simulink library "libbha_kinematic"  (R2015b)
settings: Solver=FixedStepDiscrete  StartTime=0.0  StopTime=Inf  FixedStep=0.004  RelTol=1e-3
PostLoadFcn:
  | , if any(exist('dsrtsu_mdlpostloadfcn', 'file') == [2, 3, 6]), try dsrtsu_mdlpostloadfcn('Execute', bdroot); catch fprintf('Error in PostLoadFcn (dsrtsu_mdlpostloadfcn) for model "%s":\n %s\n', bdroot, lasterr); end, end,
undefined symbols (not defined in the file or in its folder): BHA, BHASIM
libraries: libbha_kinematic x14
(part 1 of 3)
settings Model: DSRTSU_INTERNAL_RTI_VER=470  DSRTSU_INTERNAL_RTI_TYPE=rti1007  DSRTSU_INTERNAL_RTIFPGA=60  Creator=Falkenhahn  LastModifiedBy=isysfalkenhahn
settings DataIOCC: SaveFormat=Array
settings OptimizationCC: BlockReduction=off  OptimizeBlockIOStorage=off  BufferReuse=off  GlobalBufferReuse=off  ExpressionFolding=off  LocalBlockOutputs=off
settings DebuggingCC: UnderspecifiedInitializationDetection=Classic  MergeDetectMultiDrivingBlocksExec=none  SolverPrmCheckMsg=warning
settings HardwareCC: ProdBitPerPointer=32  ProdLargestAtomicFloat=None  ProdEndianess=BigEndian  ProdWordSize=32  ProdHWDeviceType=Generic->Custom  TargetIntDivRoundTo=Zero  TargetEndianess=BigEndian  TargetHWDeviceType=Generic->Custom
settings RTWCC: SystemTargetFile=rti1007.tlc  MakeCommand=make_rti  TemplateMakefile=rti1007.tmf  Description=dSPACE DS1007 Hardware Platform
settings STFCustomTargetCC: ParMdlRefBuildCompliant=on  ConcurrentExecutionCompliant=off  MatFileLogging=on  SystemTargetFile=rti1007.tlc
settings GRTTargetCC: CompOptLevelCompliant=off  ConcurrentExecutionCompliant=off  GeneratePreprocessorConditionals=Disable all  CombineOutputUpdateFcns=off  GRTInterface=on  UseToolchainInfoCompliant=off  ExtModeMexFile=noextcomm
settings ConfigComp: CovModelRefEnable=Off

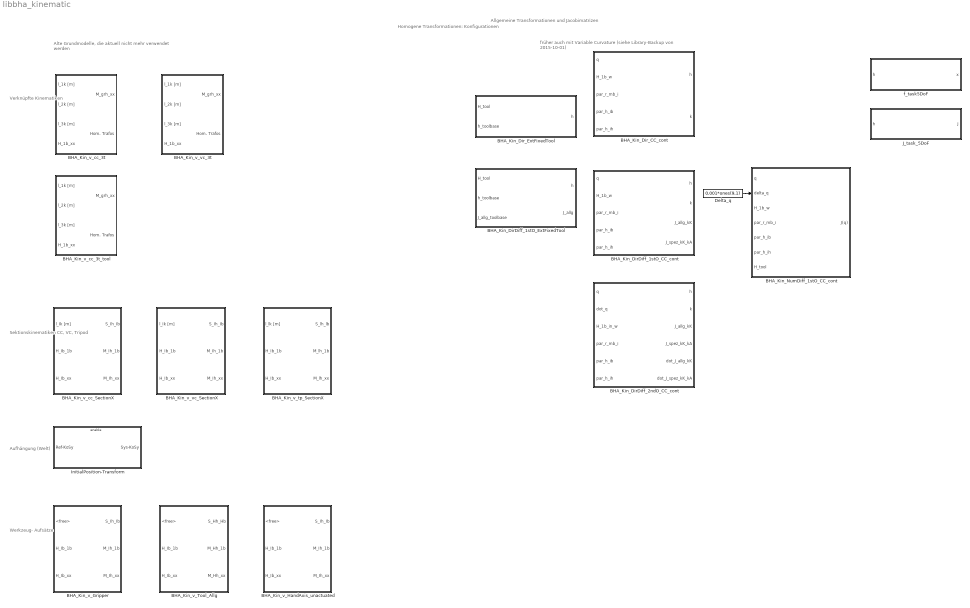
== system libbha_kinematic ==
  note: früher auch mit Variable Curvature (siehe Library-Backup von 2015-10-01)
  note: Alte Grundmodelle, die aktuell nicht mehr verwendet werden
  note: Werkzeug-
      | Aufsätze
  note: Sektionskinematiken
      | CC, VC, Tripod
  note: Verknüpfte
      | Kinematiken
  note: Aufhängung
      | (Welt)
  note: Homogene Transformationen: Konfigurationen
  note: Allgemeine Transformationen und Jacobimatrizen
  BHA_Kin_DirDiff_1stO_CC_cont : Subsystem
      settings: AttributesFormatString=|
      | Direkte Differentielle Kinematik 1. Ordnung
      | Modell: Konstante Krümmungsradien
      | Modell: Kontinuierlich biegende Aktoren
  BHA_Kin_DirDiff_1stO_ExtFixedTool : MATLAB Function  TreatAsAtomicUnit=on
  BHA_Kin_DirDiff_2ndO_CC_cont : Subsystem
      settings: AttributesFormatString=|
      | Direkte Differentielle Kinematik 2. Ordnung
      | Modell: Konstante Krümmungsradien
      | Modell: Kontinuierlich biegende Aktoren
  BHA_Kin_Dir_CC_cont : Subsystem
      settings: AttributesFormatString=|
      | Direkte Kinematik
      | Modell: Konstante Krümmungsradien
      | Modell: Kontinuierlich biegende Aktoren
  BHA_Kin_Dir_ExtFixedTool : MATLAB Function  TreatAsAtomicUnit=on
  BHA_Kin_NumDiff_1stO_CC_cont : Subsystem
      settings: AttributesFormatString=|
      | Direkte Differentielle Kinematik 1. Ordnung
      | Modell: Konstante Krümmungsradien
      | Modell: Kontinuierlich biegende Aktoren
  BHA_Kin_v_Gripper : Subsystem  mask{realorsim=real}
      mask prompts: realorsim "Parameter"
      mask init:
      | if realorsim == 1
      |     realorsimstr = 'real';
      | else
      |     realorsimstr = 'sim';
      | end
      mask TypeOptions realorsim: real | sim
      mask Display:
      | fprintf('%s\n%s','Gripper',realorsimstr)
      | port_label('input',1,'< par unused >');
      | port_label('input',2,'H_Ib_1b');
      | port_label('input',3,'H_Ib_xx');
      | 
      | port_label('output',1,'S_Ih_Ib');
      | port_label('output',2,'M_Ih_1b');
      | port_label('output',3,'M_Ih_xx');
  BHA_Kin_v_HandAxis_unactuated : Subsystem  mask{realorsim=real}
      mask prompts: realorsim "Parameter"
      mask help: -- Vorwärtskinematik der Handachse des BHAs --
      mask init:
      | if realorsim == 1
      |     realorsimstr = 'real';
      | else
      |     realorsimstr = 'sim';
      | end
      mask TypeOptions realorsim: real | sim
      mask Display:
      | fprintf('%s\n%s','H-Axis',realorsimstr)
      | port_label('input',1,'< par unused >');
      | port_label('input',2,'H_Ib_1b');
      | port_label('input',3,'H_Ib_xx');
      | 
      | port_label('output',1,'S_Ih_Ib');
      | port_label('output',2,'M_Ih_1b');
      | port_label('output',3,'M_Ih_xx');
  BHA_Kin_v_Tool_Allg : Subsystem  mask{realorsim=real}
      mask prompts: realorsim "Parameter"
      mask help: -- Vorwärtskinematik der Handachse des BHAs --
      mask init:
      | if realorsim == 1
      |     realorsimstr = 'real';
      | else
      |     realorsimstr = 'sim';
      | end
      mask TypeOptions realorsim: real | sim
      mask Display:
      | fprintf('%s\n%s','Allg. Tool',realorsimstr)
      | port_label('input',1,'< par unused >');
      | port_label('input',2,'H_Hb_1b');
      | port_label('input',3,'H_Hb_xx');
      | 
      | port_label('output',1,'S_Hh_Hb');
      | port_label('output',2,'M_Hh_1b');
      | port_label('output',3,'M_Hh_xx');
  BHA_Kin_v_cc_3t : Subsystem
  BHA_Kin_v_cc_3t_tool : Subsystem
  BHA_Kin_v_cc_SectionX : Subsystem  mask{ii=1, realorsim=real}
      mask prompts: ii "Sektionsnummer"; realorsim "Parameter"
      mask help:
      | -- Vorwärtskinematik einer Sektion des BHAs --
      |
      | Wahl der Sektionsnummer:
      | 1 = groß
      | 2 = mittel
      | 3 = klein
      mask init:
      | if realorsim == 1
      |     realorsimstr = 'real';
      | else
      |     realorsimstr = 'sim';
      | end
      mask TypeOptions ii: 1 | 2 | 3
      mask TypeOptions realorsim: real | sim
      mask Display:
      | fprintf('S #%d\n%s',ii,realorsimstr)
      | port_label('input',1,'l_Ik [m]');
      | port_label('input',2,'H_Ib_1b');
      | port_label('input',3,'H_Ib_xx');
      | 
      | port_label('output',1,'S_Ih_Ib');
      | port_label('output',2,'M_Ih_1b');
      | port_label('output',3,'M_Ih_xx');
  BHA_Kin_v_tp_SectionX : Subsystem  mask{ii=1, realorsim=real}
      mask prompts: ii "Sektionsnummer"; realorsim "Parameter"
      mask help:
      | -- Vorwärtskinematik einer Sektion des BHAs --
      |
      | Wahl der Sektionsnummer:
      | 1 = groß
      | 2 = mittel
      | 3 = klein
      mask init:
      | if realorsim == 1
      |     realorsimstr = 'real';
      | else
      |     realorsimstr = 'sim';
      | end
      mask TypeOptions ii: 1 | 2 | 3
      mask TypeOptions realorsim: real | sim
      mask Display:
      | fprintf('S #%d\n%s',ii,realorsimstr)
      | port_label('input',1,'l_Ik [m]');
      | port_label('input',2,'H_Ib_1b');
      | port_label('input',3,'H_Ib_xx');
      | 
      | port_label('output',1,'S_Ih_Ib');
      | port_label('output',2,'M_Ih_1b');
      | port_label('output',3,'M_Ih_xx');
  BHA_Kin_v_vc_3t : Subsystem
  BHA_Kin_v_vc_SectionX : Subsystem  mask{ii=1, realorsim=real}
      mask prompts: ii "Sektionsnummer"; realorsim "Parameter"
      mask help:
      | -- Vorwärtskinematik einer Sektion des BHAs --
      |
      | Wahl der Sektionsnummer:
      | 1 = groß
      | 2 = mittel
      | 3 = klein
      mask init:
      | if realorsim == 1
      |     realorsimstr = 'real';
      | else
      |     realorsimstr = 'sim';
      | end
      mask TypeOptions ii: 1 | 2 | 3
      mask TypeOptions realorsim: real | sim
      mask Display:
      | fprintf('S #%d\n%s',ii,realorsimstr)
      | port_label('input',1,'l_Ik [m]');
      | port_label('input',2,'H_Ib_1b');
      | port_label('input',3,'H_Ib_xx');
      | 
      | port_label('output',1,'S_Ih_Ib');
      | port_label('output',2,'M_Ih_1b');
      | port_label('output',3,'M_Ih_xx');
  Delta_q : Constant  Value=0.001*ones(9,1)
  InitialPosition-Transform : Subsystem  mask(Initial Position Transform){transx=2.2, transy=0, transz=0, positioning=Stehend, rotz=0}
      mask prompts: transx "Verschiebung in Welt (x) [m]"; transy "Verschiebung in Welt (y) [m]"; transz "Verschiebung in Welt (z) [m]"; positioning "Ausrichtung (Konfiguration)"; rotz "Finale Drehung um z-Achse des Balges [rad]"
      mask help:
      | Führt eine Homogene Transformation des Referenzsystems durch.
      |
      | 1. Verschiebung des Systems im Referenz-Koordinatensystem (x y z)
      | 2. Positionierung stehend (keine Transformation) oder über Kopf (Drehung um x-Achse mit 180°)
      | 3. Ausrichtung (Drehung um z-Achse des Systems, also bei hängendem System um negative Referenz-z-Achse)
      mask init:
      | % 1. Translation in Weltkoordinaten (Referenzsystem)
      | InitialHomogenTranslation = [zeros(4,3), [transx; transy; transz; 0]];
      | 
      | % 2. Umdrehen oder nicht? Über-Kopf-Hängen entspricht Rotation um x-Achse.
      | %    Dabei werden die Y- und Z-Achse umgedreht.
      | if positioning == 2 % Stehend
      |     InitialHomogenRotation = eye(4);
      |     posstr = 'stehend';
      | else % Hängend
      |     InitialHomogenRotation = [1 0 0 0; 0 -1 0 0; 0 0 -1 0; 0 0 0 1];
      |     posstr = 'hängend';
      | end
      | 
      | % 3. Rotation um die neue Z-Achse (zeigt nach unten, falls hängend).
      | InitialHomogenRotation = InitialHomogenRotation * [cos(rotz) -sin(rotz) 0 0; sin(rotz) cos(rotz) 0 0; 0 0 1 0; 0 0 0 1;];
      | 
      | 
      | %% Skript zur Initialisierung mit Matlab
      | % H_OUT = (H_IN + [zeros(4,3), [BHA.Kin.initial_translation ; 0]];
      mask TypeOptions positioning: Hängend | Stehend
      mask Display:
      | port_label('input',1,'H_ref');
      | port_label('output',1,'H_sys');
      | fprintf('Translation: [%.3g %.3g %.3g]''\nBHA %s\nRotation (z): %.1f°',transx, transy,transz,posstr,rotz*180/pi);
  J_task_5DoF : Subsystem
  f_task5DoF : Subsystem
  wires:
  Delta_q/1 -> BHA_Kin_NumDiff_1stO_CC_cont/2(delta_q)

== system libbha_kinematic/BHA_Kin_DirDiff_1stO_CC_cont ==
  q : Inport
  H_1b_w : Inport  Port=2
  par_r_mb_i : Inport  Port=3
      settings: AttributesFormatString=|
      | radialer Abstand der Aktoren
      | zur Sektionsbiegelinie pro Sektion
  par_h_ib : Inport  Port=4
      settings: AttributesFormatString=|
      | Höhe der Sektionsbasis
      | pro Sektion
  par_h_ih : Inport  Port=5
      settings: AttributesFormatString=|
      | Höhe des Sektionskopfs
      | pro Sektion
  J_general & J_specific : MATLAB Function  TreatAsAtomicUnit=on
  h : Outport
  k : Outport  Port=2
  J_allg_kK : Outport  Port=3
  J_spez_kK_kA : Outport  Port=4
  wires:
  J_general & J_specific/1(h) -> h/1
  q/1 -> J_general & J_specific/1(q)
  H_1b_w/1 -> J_general & J_specific/2(H_1b_w)
  J_general & J_specific/4(J_spez_kK_kA) -> J_spez_kK_kA/1
  J_general & J_specific/3(J_allg_kK) -> J_allg_kK/1
  J_general & J_specific/2(k) -> k/1
  par_h_ib/1 -> J_general & J_specific/4(h_ib)
  par_h_ih/1 -> J_general & J_specific/5(h_ih)
  par_r_mb_i/1 -> J_general & J_specific/3(r_i)

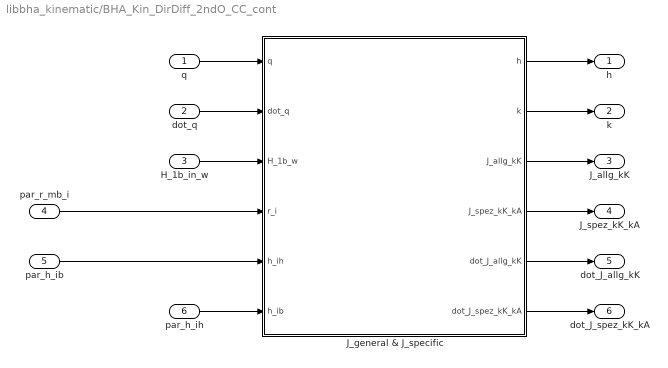
== system libbha_kinematic/BHA_Kin_DirDiff_2ndO_CC_cont ==
  q : Inport
  dot_q : Inport  Port=2
  H_1b_in_w : Inport  Port=3
  par_r_mb_i : Inport  Port=4
      settings: AttributesFormatString=|
      | radialer Abstand der Aktoren
      | zur Sektionsbiegelinie pro Sektion
  par_h_ib : Inport  Port=5
      settings: AttributesFormatString=|
      | Höhe der Sektionsbasis
      | pro Sektion
  par_h_ih : Inport  Port=6
      settings: AttributesFormatString=|
      | Höhe des Sektionskopfs
      | pro Sektion
  J_general & J_specific : MATLAB Function  TreatAsAtomicUnit=on
  h : Outport
  k : Outport  Port=2
  J_allg_kK : Outport  Port=3
  J_spez_kK_kA : Outport  Port=4
  dot_J_allg_kK : Outport  Port=5
  dot_J_spez_kK_kA : Outport  Port=6
  wires:
  dot_q/1 -> J_general & J_specific/2(dot_q)
  J_general & J_specific/6(dot_J_spez_kK_kA) -> dot_J_spez_kK_kA/1
  J_general & J_specific/5(dot_J_allg_kK) -> dot_J_allg_kK/1
  J_general & J_specific/2(k) -> k/1
  J_general & J_specific/3(J_allg_kK) -> J_allg_kK/1
  J_general & J_specific/4(J_spez_kK_kA) -> J_spez_kK_kA/1
  H_1b_in_w/1 -> J_general & J_specific/3(H_1b_w)
  q/1 -> J_general & J_specific/1(q)
  J_general & J_specific/1(h) -> h/1
  par_h_ib/1 -> J_general & J_specific/5(h_ih)
  par_h_ih/1 -> J_general & J_specific/6(h_ib)
  par_r_mb_i/1 -> J_general & J_specific/4(r_i)

== system libbha_kinematic/BHA_Kin_Dir_CC_cont ==
  q : Inport
  H_1b_w : Inport  Port=2
  par_r_mb_i : Inport  Port=3
      settings: AttributesFormatString=|
      | radialer Abstand der Aktoren
      | zur Sektionsbiegelinie pro Sektion
  par_h_ib : Inport  Port=4
      settings: AttributesFormatString=|
      | Höhe der Sektionsbasis
      | pro Sektion
  par_h_ih : Inport  Port=5
      settings: AttributesFormatString=|
      | Höhe des Sektionskopfs
      | pro Sektion
  DK_ConstCurv : MATLAB Function  TreatAsAtomicUnit=on
  h : Outport
  k : Outport  Port=2
  wires:
  DK_ConstCurv/2(k) -> k/1
  H_1b_w/1 -> DK_ConstCurv/2(H_1b_w)
  q/1 -> DK_ConstCurv/1(q)
  DK_ConstCurv/1(h) -> h/1
  par_h_ib/1 -> DK_ConstCurv/4(h_ib)
  par_h_ih/1 -> DK_ConstCurv/5(h_ih)
  par_r_mb_i/1 -> DK_ConstCurv/3(r_i)

== system libbha_kinematic/BHA_Kin_NumDiff_1stO_CC_cont ==
  q : Inport
  delta_q : Inport  Port=2
  H_1b_w : Inport  Port=3
  par_r_mb_i : Inport  Port=4
  par_h_ib : Inport  Port=5
  par_h_ih : Inport  Port=6
  H_tool : Inport  Port=7
  "Zentraler Differenzenquotient -> Jacobimatrix" : Subsystem  TreatAsAtomicUnit=on
  createForMatrix : MATLAB Function  TreatAsAtomicUnit=on
  J(q) : Outport
  wires:
  "Zentraler Differenzenquotient -> Jacobimatrix"/1(J) -> J(q)/1
  q/1 -> createForMatrix/1(q)
  createForMatrix/1(q_plus_dq) -> "Zentraler Differenzenquotient -> Jacobimatrix"/1(q+dq)
  createForMatrix/2(q_minus_dq) -> "Zentraler Differenzenquotient -> Jacobimatrix"/2(q-dq)
  createForMatrix/3(norm_dq) -> "Zentraler Differenzenquotient -> Jacobimatrix"/3(norm(dq))
  delta_q/1 -> createForMatrix/2(dq)
  H_1b_w/1 -> "Zentraler Differenzenquotient -> Jacobimatrix"/4(H_1b_w)
  par_r_mb_i/1 -> "Zentraler Differenzenquotient -> Jacobimatrix"/5(par_r_mb_i)
  par_h_ih/1 -> "Zentraler Differenzenquotient -> Jacobimatrix"/7(par_h_ih)
  par_h_ib/1 -> "Zentraler Differenzenquotient -> Jacobimatrix"/6(par_h_ib)
  H_tool/1 -> "Zentraler Differenzenquotient -> Jacobimatrix"/8(H_tool)

== system libbha_kinematic/BHA_Kin_v_Gripper ==
  <free> : Inport
  H_Ib_1b : Inport  Port=2  PortDimensions=[4 4]
  H_Ib_xx : Inport  Port=3  PortDimensions=[4 4]
  Gripper unactuated : Constant  Value=[eye(3), [0; 0; 0.060]; zeros(1,3), 1]
  Product : Product  Multiplication=Matrix(*)  RndMeth=Zero
  Product1 : Product  Multiplication=Matrix(*)  RndMeth=Zero
  Terminator : Terminator
  S_Ih_Ib : Outport  PortDimensions=[4 4]
  M_Ih_1b : Outport  Port=2  PortDimensions=[4 4]
  M_Ih_xx : Outport  Port=3  PortDimensions=[4 4]
  wires:
  <free>/1 -> Terminator/1
  Gripper unactuated/1 -> S_Ih_Ib/1, Product/2, Product1/2
  H_Ib_1b/1 -> Product1/1
  H_Ib_xx/1 -> Product/1
  Product1/1 -> M_Ih_1b/1
  Product/1 -> M_Ih_xx/1

== system libbha_kinematic/BHA_Kin_v_HandAxis_unactuated ==
  <free> : Inport
  H_Ib_1b : Inport  Port=2  PortDimensions=[4 4]
  H_Ib_xx : Inport  Port=3  PortDimensions=[4 4]
  HandAxis unactuated : Constant  Value=[eye(3), [0; 0; 0.090]; zeros(1,3), 1]
  Product : Product  Multiplication=Matrix(*)  RndMeth=Zero
  Product1 : Product  Multiplication=Matrix(*)  RndMeth=Zero
  Terminator : Terminator
  S_Ih_Ib : Outport  PortDimensions=[4 4]
  M_Ih_1b : Outport  Port=2  PortDimensions=[4 4]
  M_Ih_xx : Outport  Port=3  PortDimensions=[4 4]
  wires:
  <free>/1 -> Terminator/1
  HandAxis unactuated/1 -> S_Ih_Ib/1, Product/2, Product1/2
  H_Ib_1b/1 -> Product1/1
  H_Ib_xx/1 -> Product/1
  Product1/1 -> M_Ih_1b/1
  Product/1 -> M_Ih_xx/1

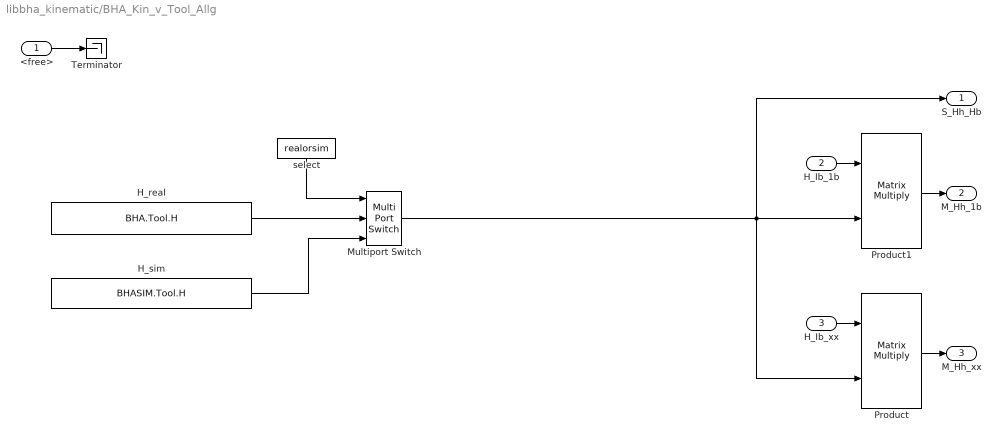
== system libbha_kinematic/BHA_Kin_v_Tool_Allg ==
  <free> : Inport
  H_Ib_1b : Inport  Port=2  PortDimensions=[4 4]
  H_Ib_xx : Inport  Port=3  PortDimensions=[4 4]
  H_real : Constant  Value=BHA.Tool.H  VectorParams1D=off
  H_sim : Constant  Value=BHASIM.Tool.H  VectorParams1D=off
  Multiport Switch : MultiPortSwitch  Inputs=2
  Product : Product  Multiplication=Matrix(*)  RndMeth=Zero
  Product1 : Product  Multiplication=Matrix(*)  RndMeth=Zero
  Terminator : Terminator
  select : Constant  Value=realorsim
  S_Hh_Hb : Outport  PortDimensions=[4 4]
  M_Hh_1b : Outport  Port=2  PortDimensions=[4 4]
  M_Hh_xx : Outport  Port=3  PortDimensions=[4 4]
  wires:
  H_sim/1 -> Multiport Switch/3
  select/1 -> Multiport Switch/1
  H_real/1 -> Multiport Switch/2
  <free>/1 -> Terminator/1
  Multiport Switch/1 -> Product1/2, S_Hh_Hb/1, Product/2
  H_Ib_1b/1 -> Product1/1
  H_Ib_xx/1 -> Product/1
  Product1/1 -> M_Hh_1b/1
  Product/1 -> M_Hh_xx/1

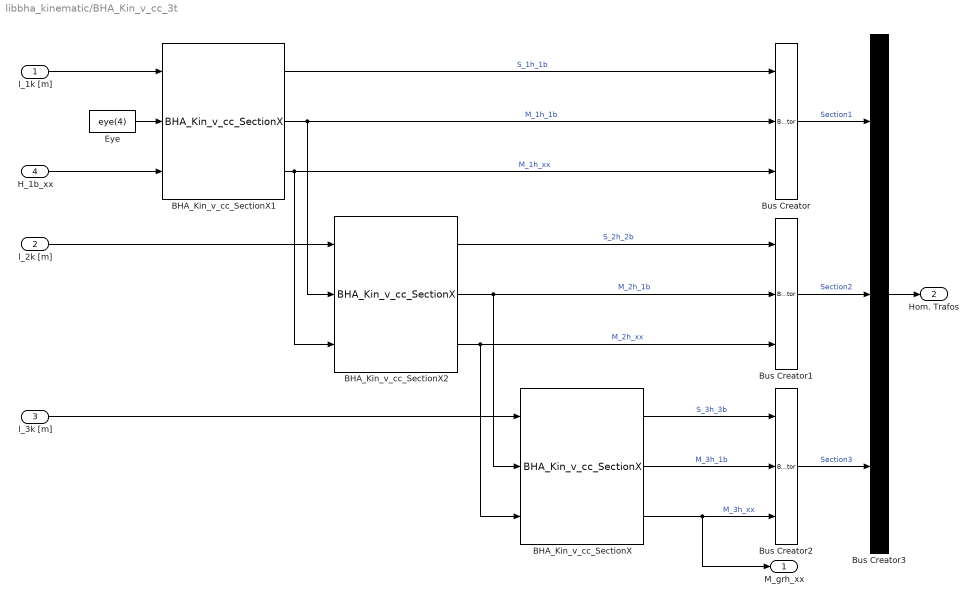
== system libbha_kinematic/BHA_Kin_v_cc_3t ==
  l_1k [m] : Inport  PortDimensions=3
  l_2k [m] : Inport  Port=2  PortDimensions=3
  l_3k [m] : Inport  Port=3  PortDimensions=3
  H_1b_xx : Inport  Port=4  PortDimensions=[4 4]
  BHA_Kin_v_cc_SectionX : libbha_kinematic/BHA_Kin_v_cc_SectionX  ii=3  realorsim=real
  BHA_Kin_v_cc_SectionX1 : libbha_kinematic/BHA_Kin_v_cc_SectionX  ii=1  realorsim=real
  BHA_Kin_v_cc_SectionX2 : libbha_kinematic/BHA_Kin_v_cc_SectionX  ii=2  realorsim=real
  Bus Creator{,1..3} (4 alike) : BusCreator  Inputs=3
  Eye : Constant  Value=eye(4)
  "M_grh_xx " : Outport
  Hom. Trafos : Outport  Port=2
  wires:
  l_1k [m]/1 -> BHA_Kin_v_cc_SectionX1/1
  Eye/1 -> BHA_Kin_v_cc_SectionX1/2
  H_1b_xx/1 -> BHA_Kin_v_cc_SectionX1/3
  l_2k [m]/1 -> BHA_Kin_v_cc_SectionX2/1
  l_3k [m]/1 -> BHA_Kin_v_cc_SectionX/1
  Bus Creator3/1 -> Hom. Trafos/1
  Bus Creator2/1 -> Bus Creator3/3  "Section3"
  Bus Creator1/1 -> Bus Creator3/2  "Section2"
  Bus Creator/1 -> Bus Creator3/1  "Section1"
  BHA_Kin_v_cc_SectionX/1 -> Bus Creator2/1  "S_3h_3b"
  BHA_Kin_v_cc_SectionX/3 -> Bus Creator2/3, "M_grh_xx "/1  "M_3h_xx"
  BHA_Kin_v_cc_SectionX/2 -> Bus Creator2/2  "M_3h_1b"
  BHA_Kin_v_cc_SectionX2/3 -> Bus Creator1/3, BHA_Kin_v_cc_SectionX/3  "M_2h_xx"
  BHA_Kin_v_cc_SectionX2/2 -> Bus Creator1/2, BHA_Kin_v_cc_SectionX/2  "M_2h_1b"
  BHA_Kin_v_cc_SectionX2/1 -> Bus Creator1/1  "S_2h_2b"
  BHA_Kin_v_cc_SectionX1/1 -> Bus Creator/1  "S_1h_1b"
  BHA_Kin_v_cc_SectionX1/2 -> Bus Creator/2, BHA_Kin_v_cc_SectionX2/2  "M_1h_1b"
  BHA_Kin_v_cc_SectionX1/3 -> Bus Creator/3, BHA_Kin_v_cc_SectionX2/3  "M_1h_xx"

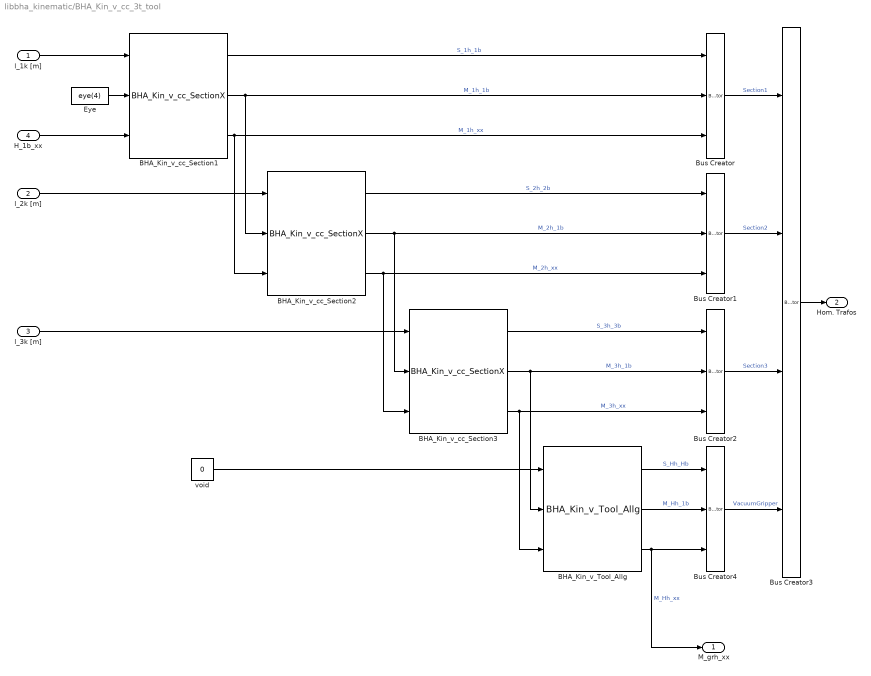
== system libbha_kinematic/BHA_Kin_v_cc_3t_tool ==
  l_1k [m] : Inport  PortDimensions=3
  l_2k [m] : Inport  Port=2  PortDimensions=3
  l_3k [m] : Inport  Port=3  PortDimensions=3
  H_1b_xx : Inport  Port=4  PortDimensions=[4 4]
  BHA_Kin_v_Tool_Allg : libbha_kinematic/BHA_Kin_v_Tool_Allg  realorsim=real
  BHA_Kin_v_cc_Section1 : libbha_kinematic/BHA_Kin_v_cc_SectionX  ii=1  realorsim=real
  BHA_Kin_v_cc_Section2 : libbha_kinematic/BHA_Kin_v_cc_SectionX  ii=2  realorsim=real
  BHA_Kin_v_cc_Section3 : libbha_kinematic/BHA_Kin_v_cc_SectionX  ii=3  realorsim=real
  Bus Creator{,1..2,4} (4 alike) : BusCreator  Inputs=3
  Bus Creator3 : BusCreator  Inputs=4
  Eye : Constant  Value=eye(4)
  void : Constant  Value=0
  "M_grh_xx " : Outport
  Hom. Trafos : Outport  Port=2
  wires:
  BHA_Kin_v_cc_Section1/3 -> BHA_Kin_v_cc_Section2/3, Bus Creator/3  "M_1h_xx"
  BHA_Kin_v_cc_Section1/2 -> BHA_Kin_v_cc_Section2/2, Bus Creator/2  "M_1h_1b"
  BHA_Kin_v_cc_Section1/1 -> Bus Creator/1  "S_1h_1b"
  BHA_Kin_v_cc_Section2/1 -> Bus Creator1/1  "S_2h_2b"
  BHA_Kin_v_cc_Section2/2 -> BHA_Kin_v_cc_Section3/2, Bus Creator1/2  "M_2h_1b"
  BHA_Kin_v_cc_Section2/3 -> BHA_Kin_v_cc_Section3/3, Bus Creator1/3  "M_2h_xx"
  BHA_Kin_v_cc_Section3/2 -> BHA_Kin_v_Tool_Allg/2, Bus Creator2/2  "M_3h_1b"
  BHA_Kin_v_cc_Section3/3 -> BHA_Kin_v_Tool_Allg/3, Bus Creator2/3  "M_3h_xx"
  BHA_Kin_v_cc_Section3/1 -> Bus Creator2/1  "S_3h_3b"
  Bus Creator/1 -> Bus Creator3/1  "Section1"
  Bus Creator1/1 -> Bus Creator3/2  "Section2"
  Bus Creator2/1 -> Bus Creator3/3  "Section3"
  Bus Creator3/1 -> Hom. Trafos/1
  l_3k [m]/1 -> BHA_Kin_v_cc_Section3/1
  l_2k [m]/1 -> BHA_Kin_v_cc_Section2/1
  H_1b_xx/1 -> BHA_Kin_v_cc_Section1/3
  Eye/1 -> BHA_Kin_v_cc_Section1/2
  l_1k [m]/1 -> BHA_Kin_v_cc_Section1/1
  void/1 -> BHA_Kin_v_Tool_Allg/1
  BHA_Kin_v_Tool_Allg/1 -> Bus Creator4/1  "S_Hh_Hb"
  BHA_Kin_v_Tool_Allg/2 -> Bus Creator4/2  "M_Hh_1b"
  BHA_Kin_v_Tool_Allg/3 -> "M_grh_xx "/1, Bus Creator4/3  "M_Hh_xx"
  Bus Creator4/1 -> Bus Creator3/4  "VacuumGripper"

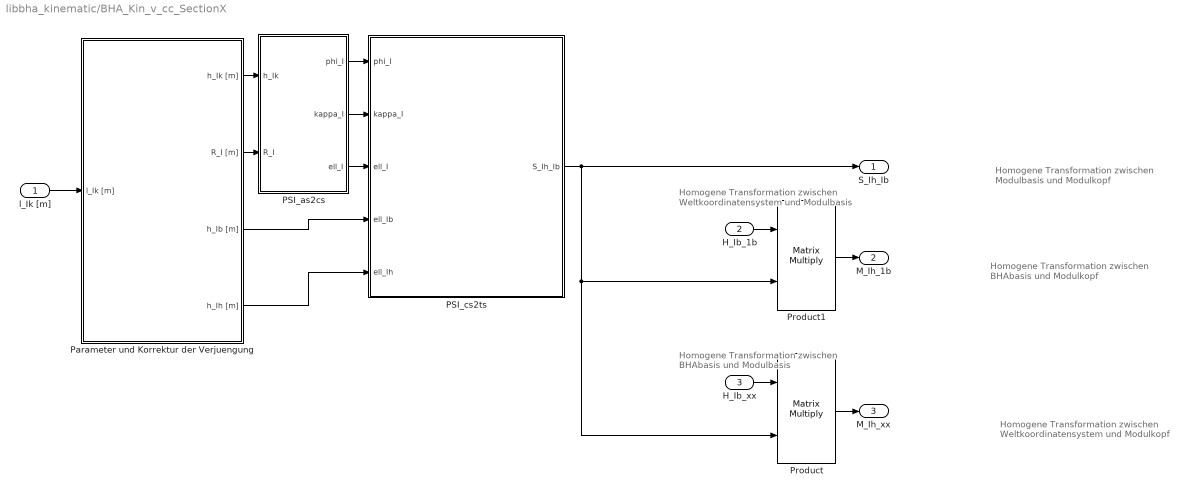
== system libbha_kinematic/BHA_Kin_v_cc_SectionX ==
  note: Homogene Transformation zwischen
      | Weltkoordinatensystem und Modulbasis
  note: Homogene Transformation zwischen
      | BHAbasis und Modulbasis
  note: Homogene Transformation zwischen
      | Weltkoordinatensystem und Modulkopf
  note: Homogene Transformation zwischen
      | BHAbasis und Modulkopf
  note: Homogene Transformation zwischen
      | Modulbasis und Modulkopf
  l_Ik [m] : Inport  PortDimensions=3
  H_Ib_1b : Inport  Port=2  PortDimensions=[4 4]
  H_Ib_xx : Inport  Port=3  PortDimensions=[4 4]
  PSI_as2cs : Subsystem
  PSI_cs2ts : MATLAB Function  TreatAsAtomicUnit=on
  Parameter und Korrektur der Verjuengung : Subsystem
  Product : Product  Multiplication=Matrix(*)  RndMeth=Zero
  Product1 : Product  Multiplication=Matrix(*)  RndMeth=Zero
  S_Ih_Ib : Outport  PortDimensions=[4 4]
  M_Ih_1b : Outport  Port=2  PortDimensions=[4 4]
  M_Ih_xx : Outport  Port=3  PortDimensions=[4 4]
  wires:
  Product/1 -> M_Ih_xx/1
  Product1/1 -> M_Ih_1b/1
  H_Ib_xx/1 -> Product/1
  H_Ib_1b/1 -> Product1/1
  PSI_cs2ts/1(S_Ih_Ib) -> Product1/2, Product/2, S_Ih_Ib/1
  l_Ik [m]/1 -> Parameter und Korrektur der Verjuengung/1(l_Ik [m])
  Parameter und Korrektur der Verjuengung/4(h_Ih [m]) -> PSI_cs2ts/5(ell_Ih)
  Parameter und Korrektur der Verjuengung/3(h_Ib [m]) -> PSI_cs2ts/4(ell_Ib)
  PSI_as2cs/3(ell_I) -> PSI_cs2ts/3(ell_I)
  PSI_as2cs/2(kappa_I) -> PSI_cs2ts/2(kappa_I)
  PSI_as2cs/1(phi_I) -> PSI_cs2ts/1(phi_I)
  Parameter und Korrektur der Verjuengung/2(R_I [m]) -> PSI_as2cs/2(R_I)
  Parameter und Korrektur der Verjuengung/1(h_Ik [m]) -> PSI_as2cs/1(h_Ik)

== system libbha_kinematic/BHA_Kin_v_tp_SectionX ==
  l_lk [m] : Inport  PortDimensions=3
  H_Ib_1b : Inport  Port=2  PortDimensions=[4 4]
  H_Ib_xx : Inport  Port=3  PortDimensions=[4 4]
  Kin_v_Modul : MATLAB Function  TreatAsAtomicUnit=on
  Parameter und Korrektur der Verjuengung : Subsystem
  Product : Product  Multiplication=Matrix(*)  RndMeth=Zero
  Product1 : Product  Multiplication=Matrix(*)  RndMeth=Zero
  S_lh_lb : Outport  PortDimensions=[4 4]
  M_lh_1b : Outport  Port=2  PortDimensions=[4 4]
  M_lh_xx : Outport  Port=3  PortDimensions=[4 4]
  wires:
  Parameter und Korrektur der Verjuengung/7(theta_I) -> Kin_v_Modul/7(theta_I)
  Parameter und Korrektur der Verjuengung/6(l_Ih) -> Kin_v_Modul/6(l_Ih)
  Parameter und Korrektur der Verjuengung/5(l_Ib) -> Kin_v_Modul/5(l_Ib)
  Parameter und Korrektur der Verjuengung/4(a_Im) -> Kin_v_Modul/4(a_Im)
  Parameter und Korrektur der Verjuengung/3(a_I0) -> Kin_v_Modul/3(a_I0)
  Parameter und Korrektur der Verjuengung/2(m_I) -> Kin_v_Modul/2(m_I)
  Parameter und Korrektur der Verjuengung/1(l_Ik [m] out) -> Kin_v_Modul/1(l_Ik)
  l_lk [m]/1 -> Parameter und Korrektur der Verjuengung/1(l_Ik [m])
  Kin_v_Modul/1(S_lh_lb) -> S_lh_lb/1, Product/2, Product1/2
  H_Ib_1b/1 -> Product1/1
  H_Ib_xx/1 -> Product/1
  Product1/1 -> M_lh_1b/1
  Product/1 -> M_lh_xx/1

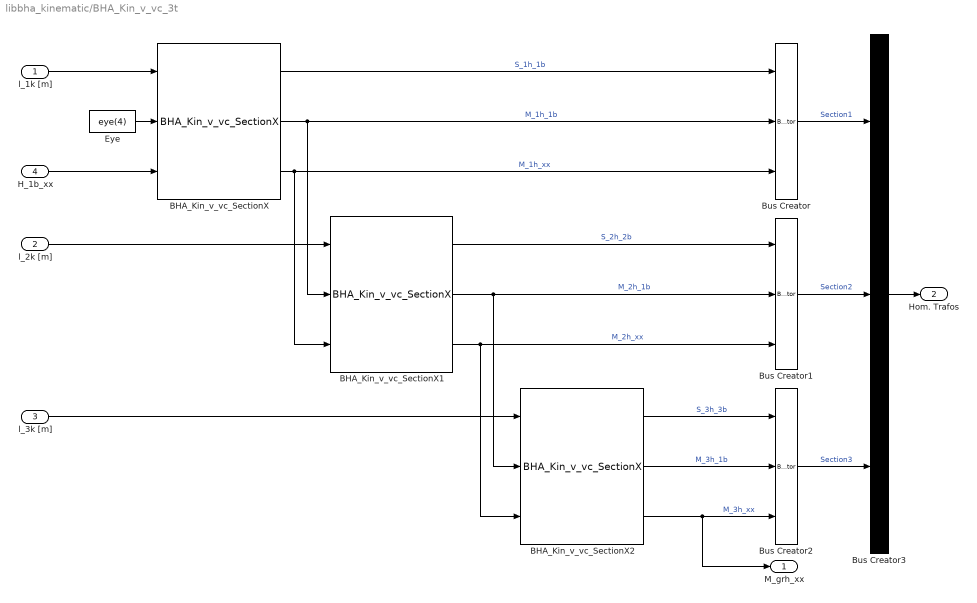
== system libbha_kinematic/BHA_Kin_v_vc_3t ==
  l_1k [m] : Inport  PortDimensions=3
  l_2k [m] : Inport  Port=2  PortDimensions=3
  l_3k [m] : Inport  Port=3  PortDimensions=3
  H_1b_xx : Inport  Port=4  PortDimensions=[4 4]
  BHA_Kin_v_vc_SectionX : libbha_kinematic/BHA_Kin_v_vc_SectionX  ii=1  realorsim=real
  BHA_Kin_v_vc_SectionX1 : libbha_kinematic/BHA_Kin_v_vc_SectionX  ii=2  realorsim=real
  BHA_Kin_v_vc_SectionX2 : libbha_kinematic/BHA_Kin_v_vc_SectionX  ii=3  realorsim=real
  Bus Creator{,1..3} (4 alike) : BusCreator  Inputs=3
  Eye : Constant  Value=eye(4)
  "M_grh_xx " : Outport
  Hom. Trafos : Outport  Port=2
  wires:
  BHA_Kin_v_vc_SectionX/3 -> BHA_Kin_v_vc_SectionX1/3, Bus Creator/3  "M_1h_xx"
  BHA_Kin_v_vc_SectionX/2 -> BHA_Kin_v_vc_SectionX1/2, Bus Creator/2  "M_1h_1b"
  BHA_Kin_v_vc_SectionX/1 -> Bus Creator/1  "S_1h_1b"
  BHA_Kin_v_vc_SectionX1/1 -> Bus Creator1/1  "S_2h_2b"
  BHA_Kin_v_vc_SectionX1/2 -> BHA_Kin_v_vc_SectionX2/2, Bus Creator1/2  "M_2h_1b"
  BHA_Kin_v_vc_SectionX1/3 -> BHA_Kin_v_vc_SectionX2/3, Bus Creator1/3  "M_2h_xx"
  BHA_Kin_v_vc_SectionX2/2 -> Bus Creator2/2  "M_3h_1b"
  BHA_Kin_v_vc_SectionX2/3 -> "M_grh_xx "/1, Bus Creator2/3  "M_3h_xx"
  BHA_Kin_v_vc_SectionX2/1 -> Bus Creator2/1  "S_3h_3b"
  Bus Creator/1 -> Bus Creator3/1  "Section1"
  Bus Creator1/1 -> Bus Creator3/2  "Section2"
  Bus Creator2/1 -> Bus Creator3/3  "Section3"
  Bus Creator3/1 -> Hom. Trafos/1
  l_3k [m]/1 -> BHA_Kin_v_vc_SectionX2/1
  l_2k [m]/1 -> BHA_Kin_v_vc_SectionX1/1
  H_1b_xx/1 -> BHA_Kin_v_vc_SectionX/3
  Eye/1 -> BHA_Kin_v_vc_SectionX/2
  l_1k [m]/1 -> BHA_Kin_v_vc_SectionX/1

== system libbha_kinematic/BHA_Kin_v_vc_SectionX ==
  note: Homogene Transformation zwischen
      | Weltkoordinatensystem und Modulbasis
  note: Homogene Transformation zwischen
      | BHAbasis und Modulbasis
  note: Homogene Transformation zwischen
      | Weltkoordinatensystem und Modulkopf
  note: Homogene Transformation zwischen
      | BHAbasis und Modulkopf
  note: Homogene Transformation zwischen
      | Modulbasis und Modulkopf
  l_Ik [m] : Inport  PortDimensions=3
  H_Ib_1b : Inport  Port=2  PortDimensions=[4 4]
  H_Ib_xx : Inport  Port=3  PortDimensions=[4 4]
  Parameter und Korrektur der Verjuengung : Subsystem
  Product : Product  Multiplication=Matrix(*)  RndMeth=Zero
  Product1 : Product  Multiplication=Matrix(*)  RndMeth=Zero
  S_RIj_R1b : Terminator
  Section-Kinematics : MATLAB Function  TreatAsAtomicUnit=on
  S_Ih_Ib : Outport  PortDimensions=[4 4]
  M_Ih_1b : Outport  Port=2  PortDimensions=[4 4]
  M_Ih_xx : Outport  Port=3  PortDimensions=[4 4]
  wires:
  Section-Kinematics/2(S_RIj_RIb) -> S_RIj_R1b/1
  Parameter und Korrektur der Verjuengung/5(theta_I) -> Section-Kinematics/5(theta_I)
  Parameter und Korrektur der Verjuengung/4(l_Ih) -> Section-Kinematics/4(l_Ih)
  Parameter und Korrektur der Verjuengung/3(l_Ib) -> Section-Kinematics/3(l_Ib)
  Parameter und Korrektur der Verjuengung/2(d_lj) -> Section-Kinematics/2(d_Ij)
  Parameter und Korrektur der Verjuengung/1(l_Ik [m]_out) -> Section-Kinematics/1(l_Ik)
  Product/1 -> M_Ih_xx/1
  Product1/1 -> M_Ih_1b/1
  H_Ib_xx/1 -> Product/1
  H_Ib_1b/1 -> Section-Kinematics/6(T_KImb_Ib), Product1/1
  Section-Kinematics/1(S_RIh_RIb) -> Product1/2, Product/2, S_Ih_Ib/1
  l_Ik [m]/1 -> Parameter und Korrektur der Verjuengung/1(l_Ik [m])

== system libbha_kinematic/InitialPosition-Transform ==
  Ref-KoSy : Inport  PortDimensions=[4 4]
  Enable : EnablePort
  Add : Sum
  Product1 : Product  Multiplication=Matrix(*)  RndMeth=Zero
  Rotation : Constant  Value=InitialHomogenRotation
  Translation : Constant  Value=InitialHomogenTranslation
  Sys-KoSy : Outport  PortDimensions=[4 4]  InitialOutput=eye(4)
  wires:
  Product1/1 -> Sys-KoSy/1
  Rotation/1 -> Product1/2
  Add/1 -> Product1/1
  Ref-KoSy/1 -> Add/1
  Translation/1 -> Add/2

== system libbha_kinematic/J_task_5DoF ==
  h : Inport
  J_task_5DoF : MATLAB Function  TreatAsAtomicUnit=on
  J : Outport
  wires:
  J_task_5DoF/1(J) -> J/1
  h/1 -> J_task_5DoF/1(h)

== system libbha_kinematic/f_task5DoF ==
  h : Inport
  f_task5DoF : MATLAB Function  TreatAsAtomicUnit=on
  x : Outport
  wires:
  f_task5DoF/1(x) -> x/1
  h/1 -> f_task5DoF/1(h)

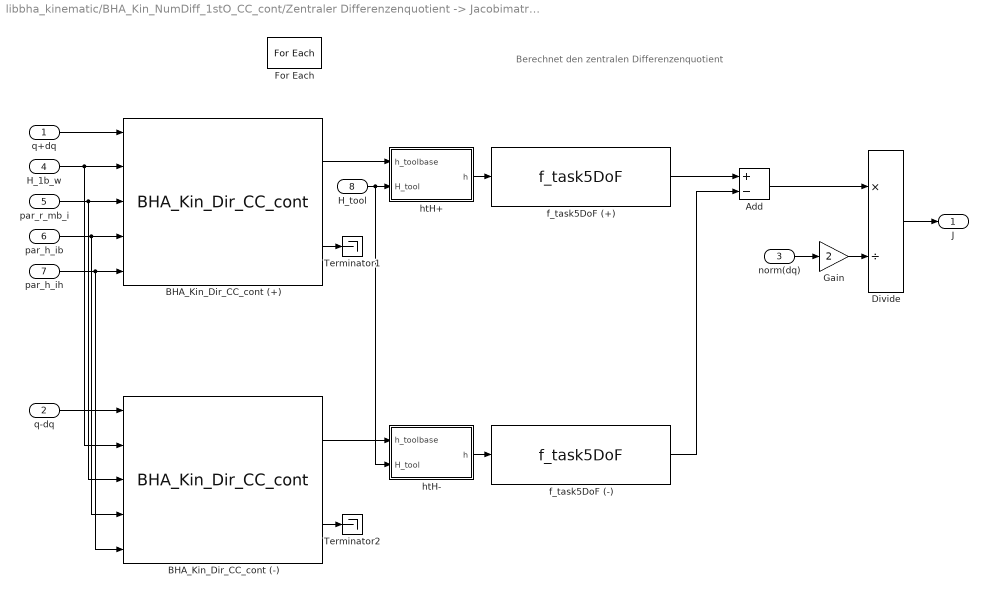
== system libbha_kinematic/BHA_Kin_NumDiff_1stO_CC_cont/Zentraler Differenzenquotient -> Jacobimatrix ==
  note: Berechnet den zentralen Differenzenquotient
  q+dq : Inport  Partition=on  PartitionDimension=3  PartitionWidth=1
  q-dq : Inport  Port=2  Partition=on  PartitionDimension=3  PartitionWidth=1
  norm(dq) : Inport  Port=3  Partition=on  PartitionDimension=3  PartitionWidth=1
  H_1b_w : Inport  Port=4
  par_r_mb_i : Inport  Port=5
  par_h_ib : Inport  Port=6
  par_h_ih : Inport  Port=7
  H_tool : Inport  Port=8
  Add : Sum  Inputs=+-
  BHA_Kin_Dir_CC_cont (+) : libbha_kinematic/BHA_Kin_Dir_CC_cont
      settings: AttributesFormatString=|
      | Direkte Kinematik
      | Modell: Konstante Krümmungsradien
      | Modell: Kontinuierlich biegende Aktoren
  BHA_Kin_Dir_CC_cont (-) : libbha_kinematic/BHA_Kin_Dir_CC_cont
      settings: AttributesFormatString=|
      | Direkte Kinematik
      | Modell: Konstante Krümmungsradien
      | Modell: Kontinuierlich biegende Aktoren
  Divide : Product  Inputs=*/
  For Each : ForEach  DisableCoverage=on  IndexMode=One-based
  Gain : Gain  Gain=2
  Terminator1 : Terminator
  Terminator2 : Terminator
  f_task5DoF (+) : libbha_kinematic/f_task5DoF
  f_task5DoF (-) : libbha_kinematic/f_task5DoF
  htH+ : MATLAB Function  TreatAsAtomicUnit=on
  htH- : MATLAB Function  TreatAsAtomicUnit=on
  J : Outport  ConcatenationDimension=2
  wires:
  norm(dq)/1 -> Gain/1
  f_task5DoF (-)/1 -> Add/2
  f_task5DoF (+)/1 -> Add/1
  Divide/1 -> J/1
  Add/1 -> Divide/1
  Gain/1 -> Divide/2
  BHA_Kin_Dir_CC_cont (+)/2 -> Terminator1/1
  htH-/1(h) -> f_task5DoF (-)/1
  BHA_Kin_Dir_CC_cont (-)/2 -> Terminator2/1
  q+dq/1 -> BHA_Kin_Dir_CC_cont (+)/1
  q-dq/1 -> BHA_Kin_Dir_CC_cont (-)/1
  H_1b_w/1 -> BHA_Kin_Dir_CC_cont (-)/2, BHA_Kin_Dir_CC_cont (+)/2
  par_r_mb_i/1 -> BHA_Kin_Dir_CC_cont (-)/3, BHA_Kin_Dir_CC_cont (+)/3
  par_h_ib/1 -> BHA_Kin_Dir_CC_cont (-)/4, BHA_Kin_Dir_CC_cont (+)/4
  par_h_ih/1 -> BHA_Kin_Dir_CC_cont (-)/5, BHA_Kin_Dir_CC_cont (+)/5
  htH+/1(h) -> f_task5DoF (+)/1
  BHA_Kin_Dir_CC_cont (+)/1 -> htH+/1(h_toolbase)
  BHA_Kin_Dir_CC_cont (-)/1 -> htH-/1(h_toolbase)
  H_tool/1 -> htH-/2(H_tool), htH+/2(H_tool)

== system libbha_kinematic/BHA_Kin_v_cc_SectionX/PSI_as2cs ==
  h_Ik : Inport
  R_I : Inport  Port=2
  ell : Subsystem
  kappa : Subsystem
  phi : Subsystem
  phi_I : Outport
  kappa_I : Outport  Port=2
  ell_I : Outport  Port=3
  wires:
  R_I/1 -> kappa/2(R_I)
  ell/1(ell_I) -> ell_I/1
  kappa/1(kappa_I) -> kappa_I/1
  phi/1(phi_I) -> phi_I/1
  h_Ik/1 -> ell/1(h_Ik), kappa/1(h_Ik), phi/1(h_Ik)

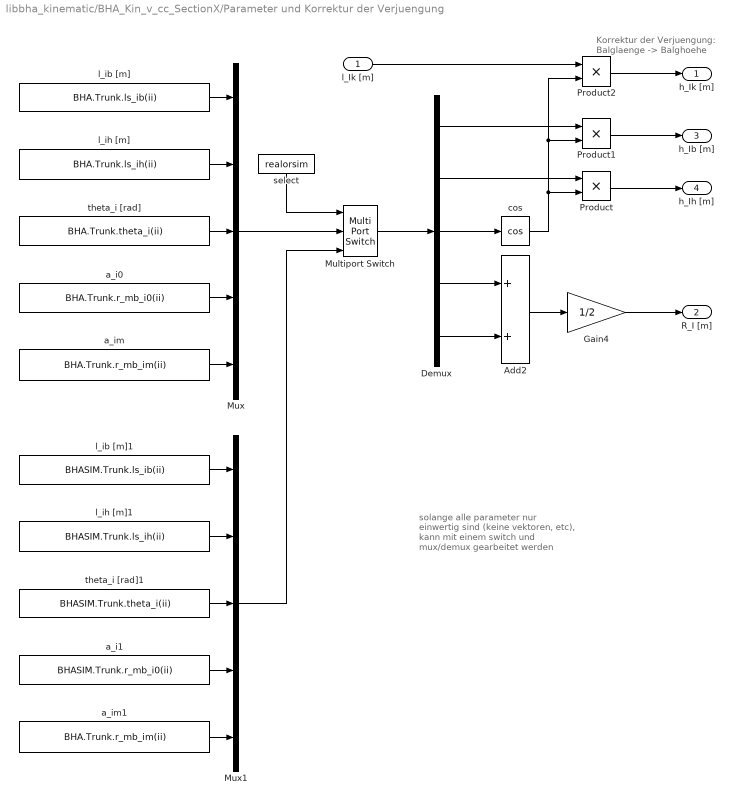
== system libbha_kinematic/BHA_Kin_v_cc_SectionX/Parameter und Korrektur der Verjuengung ==
  note: Korrektur der Verjuengung:
      | Balglaenge -> Balghoehe
  note: solange alle parameter nur einwertig
      | sind  (keine vektoren, etc),
      | kann mit einem switch und
      | mux/demux gearbeitet werden
  l_Ik [m] : Inport
  Add2 : Sum
  Demux : Demux  Outputs=5
  Gain4 : Gain  Gain=1/2
  Multiport Switch : MultiPortSwitch  Inputs=2
  Mux : Mux  Inputs=5
  Mux1 : Mux  Inputs=5
  Product : Product  RndMeth=Zero
  Product1 : Product  RndMeth=Zero
  Product2 : Product  RndMeth=Zero
  a_i0 : Constant  Value=BHA.Trunk.r_mb_i0(ii)  VectorParams1D=off
  a_i1 : Constant  Value=BHASIM.Trunk.r_mb_i0(ii)  VectorParams1D=off
  a_im : Constant  Value=BHA.Trunk.r_mb_im(ii)  VectorParams1D=off
  a_im1 : Constant  Value=BHA.Trunk.r_mb_im(ii)  VectorParams1D=off
  cos : Trigonometry  Operator=cos
  l_ib [m] : Constant  Value=BHA.Trunk.ls_ib(ii)  VectorParams1D=off
  l_ib [m]1 : Constant  Value=BHASIM.Trunk.ls_ib(ii)  VectorParams1D=off
  l_ih [m] : Constant  Value=BHA.Trunk.ls_ih(ii)  VectorParams1D=off
  l_ih [m]1 : Constant  Value=BHASIM.Trunk.ls_ih(ii)  VectorParams1D=off
  select : Constant  Value=realorsim
  theta_i [rad] : Constant  Value=BHA.Trunk.theta_i(ii)  VectorParams1D=off
  theta_i [rad]1 : Constant  Value=BHASIM.Trunk.theta_i(ii)  VectorParams1D=off
  h_Ik [m] : Outport
  R_I [m] : Outport  Port=2
  h_Ib [m] : Outport  Port=3
  h_Ih [m] : Outport  Port=4
  wires:
  select/1 -> Multiport Switch/1
  Mux1/1 -> Multiport Switch/3
  Multiport Switch/1 -> Demux/1
  Mux/1 -> Multiport Switch/2
  Demux/5 -> Add2/2
  Demux/4 -> Add2/1
  Demux/3 -> cos/1
  Demux/2 -> Product/1
  Demux/1 -> Product1/1
  a_im1/1 -> Mux1/5
  a_i1/1 -> Mux1/4
  theta_i [rad]1/1 -> Mux1/3
  l_ih [m]1/1 -> Mux1/2
  l_ib [m]1/1 -> Mux1/1
  a_im/1 -> Mux/5
  a_i0/1 -> Mux/4
  theta_i [rad]/1 -> Mux/3
  l_ih [m]/1 -> Mux/2
  l_ib [m]/1 -> Mux/1
  Gain4/1 -> R_I [m]/1
  Add2/1 -> Gain4/1
  Product/1 -> h_Ih [m]/1
  Product1/1 -> h_Ib [m]/1
  Product2/1 -> h_Ik [m]/1
  l_Ik [m]/1 -> Product2/1
  cos/1 -> Product2/2, Product1/2, Product/2

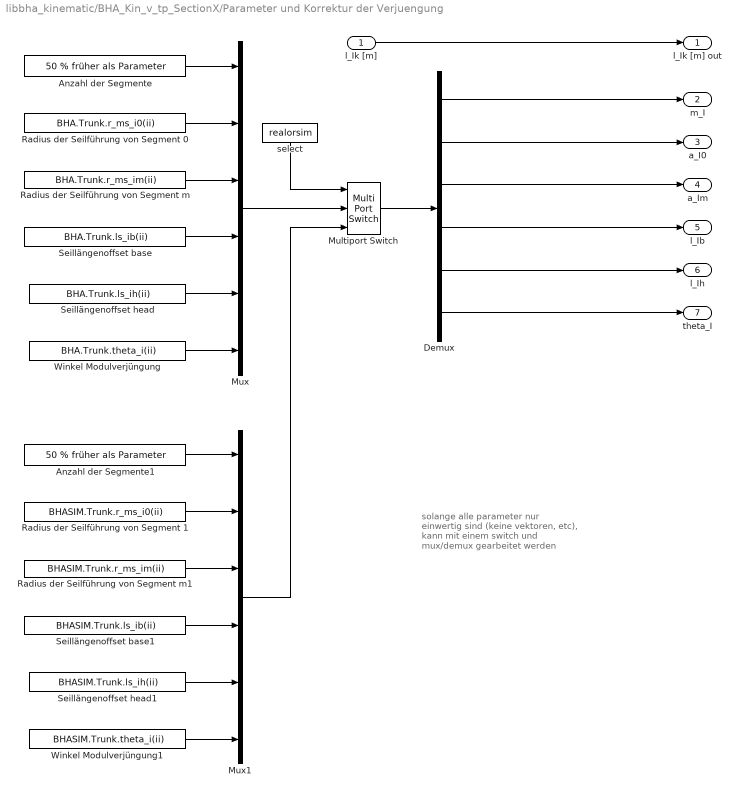
== system libbha_kinematic/BHA_Kin_v_tp_SectionX/Parameter und Korrektur der Verjuengung ==
  note: solange alle parameter nur einwertig
      | sind  (keine vektoren, etc),
      | kann mit einem switch und
      | mux/demux gearbeitet werden
  l_Ik [m] : Inport
  Anzahl der Segmente : Constant  Value=50 % früher als Parameter
  Anzahl der Segmente1 : Constant  Value=50 % früher als Parameter
  Demux : Demux  Outputs=6
  Multiport Switch : MultiPortSwitch  Inputs=2
  Mux : Mux  Inputs=6
  Mux1 : Mux  Inputs=6
  Radius der Seilführung von Segment 0 : Constant  Value=BHA.Trunk.r_ms_i0(ii)
  Radius der Seilführung von Segment 1 : Constant  Value=BHASIM.Trunk.r_ms_i0(ii)
  Radius der Seilführung von Segment m : Constant  Value=BHA.Trunk.r_ms_im(ii)
  Radius der Seilführung von Segment m1 : Constant  Value=BHASIM.Trunk.r_ms_im(ii)
  Seillängenoffset base : Constant  Value=BHA.Trunk.ls_ib(ii)
  Seillängenoffset base1 : Constant  Value=BHASIM.Trunk.ls_ib(ii)
  Seillängenoffset head : Constant  Value=BHA.Trunk.ls_ih(ii)
  Seillängenoffset head1 : Constant  Value=BHASIM.Trunk.ls_ih(ii)
  Winkel Modulverjüngung : Constant  Value=BHA.Trunk.theta_i(ii)
  Winkel Modulverjüngung1 : Constant  Value=BHASIM.Trunk.theta_i(ii)
  select : Constant  Value=realorsim
  l_Ik [m] out : Outport
  m_I : Outport  Port=2
  a_I0 : Outport  Port=3
  a_Im : Outport  Port=4
  l_Ib : Outport  Port=5
  l_Ih : Outport  Port=6
  theta_I : Outport  Port=7
  wires:
  Demux/6 -> theta_I/1
  Demux/5 -> l_Ih/1
  Demux/4 -> l_Ib/1
  Demux/3 -> a_Im/1
  Demux/2 -> a_I0/1
  Demux/1 -> m_I/1
  l_Ik [m]/1 -> l_Ik [m] out/1
  Mux1/1 -> Multiport Switch/3
  Winkel Modulverjüngung1/1 -> Mux1/6
  Seillängenoffset head1/1 -> Mux1/5
  Seillängenoffset base1/1 -> Mux1/4
  Radius der Seilführung von Segment m1/1 -> Mux1/3
  Radius der Seilführung von Segment 1/1 -> Mux1/2
  Anzahl der Segmente1/1 -> Mux1/1
  Winkel Modulverjüngung/1 -> Mux/6
  Seillängenoffset head/1 -> Mux/5
  Seillängenoffset base/1 -> Mux/4
  Radius der Seilführung von Segment m/1 -> Mux/3
  Radius der Seilführung von Segment 0/1 -> Mux/2
  Anzahl der Segmente/1 -> Mux/1
  Mux/1 -> Multiport Switch/2
  Multiport Switch/1 -> Demux/1
  select/1 -> Multiport Switch/1

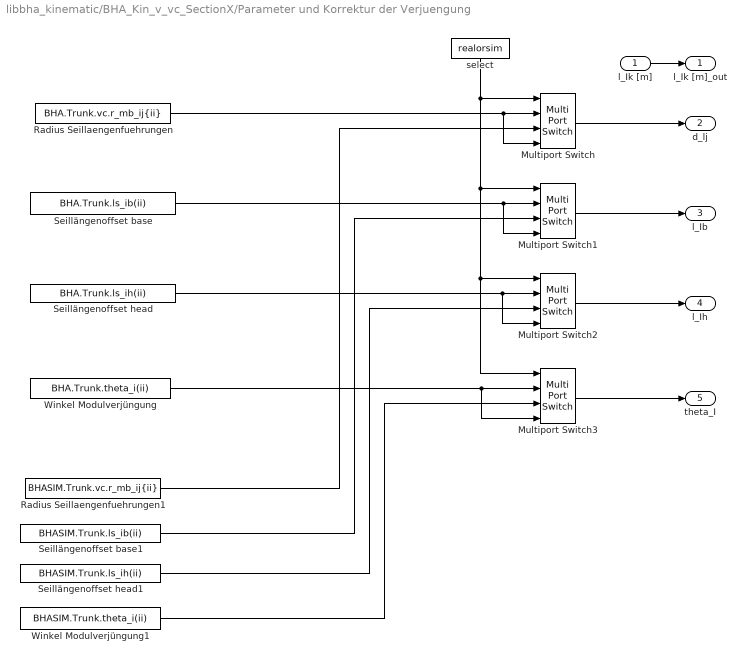
== system libbha_kinematic/BHA_Kin_v_vc_SectionX/Parameter und Korrektur der Verjuengung ==
  l_Ik [m] : Inport
  Multiport Switch{,1..3} (4 alike) : MultiPortSwitch  Inputs=2  DataPortForDefault=Additional data port
  Radius Seillaengenfuehrungen : Constant  Value=BHA.Trunk.vc.r_mb_ij{ii}
  Radius Seillaengenfuehrungen1 : Constant  Value=BHASIM.Trunk.vc.r_mb_ij{ii}
  Seillängenoffset base : Constant  Value=BHA.Trunk.ls_ib(ii)
  Seillängenoffset base1 : Constant  Value=BHASIM.Trunk.ls_ib(ii)
  Seillängenoffset head : Constant  Value=BHA.Trunk.ls_ih(ii)
  Seillängenoffset head1 : Constant  Value=BHASIM.Trunk.ls_ih(ii)
  Winkel Modulverjüngung : Constant  Value=BHA.Trunk.theta_i(ii)
  Winkel Modulverjüngung1 : Constant  Value=BHASIM.Trunk.theta_i(ii)
  select : Constant  Value=realorsim
  l_Ik [m]_out : Outport
  d_lj : Outport  Port=2
  l_Ib : Outport  Port=3
  l_Ih : Outport  Port=4
  theta_I : Outport  Port=5
  wires:
  Winkel Modulverjüngung/1 -> Multiport Switch3/2, Multiport Switch3/4
  Seillängenoffset head/1 -> Multiport Switch2/2, Multiport Switch2/4
  Seillängenoffset base/1 -> Multiport Switch1/2, Multiport Switch1/4
  Multiport Switch3/1 -> theta_I/1
  Multiport Switch2/1 -> l_Ih/1
  Multiport Switch1/1 -> l_Ib/1
  Radius Seillaengenfuehrungen/1 -> Multiport Switch/2, Multiport Switch/4
  Multiport Switch/1 -> d_lj/1
  l_Ik [m]/1 -> l_Ik [m]_out/1
  Winkel Modulverjüngung1/1 -> Multiport Switch3/3
  Seillängenoffset head1/1 -> Multiport Switch2/3
  Seillängenoffset base1/1 -> Multiport Switch1/3
  Radius Seillaengenfuehrungen1/1 -> Multiport Switch/3
  select/1 -> Multiport Switch/1, Multiport Switch1/1, Multiport Switch3/1, Multiport Switch2/1

== system libbha_kinematic/BHA_Kin_v_cc_SectionX/PSI_as2cs/ell ==
  h_Ik : Inport
  Add1 : Sum  Inputs=+++
  Gain1 : Gain  Gain=1/3
  Selector3 : Selector  InputPortWidth=3  IndexOptions=Index vector (dialog)  Indices=3  OutputSizes=1
  Selector4 : Selector  InputPortWidth=3  IndexOptions=Index vector (dialog)  Indices=2  OutputSizes=1
  Selector5 : Selector  InputPortWidth=3  IndexOptions=Index vector (dialog)  Indices=1  OutputSizes=1
  ell_I : Outport
  wires:
  Selector3/1 -> Add1/3
  Selector4/1 -> Add1/2
  Selector5/1 -> Add1/1
  h_Ik/1 -> Selector3/1, Selector4/1, Selector5/1
  Add1/1 -> Gain1/1
  Gain1/1 -> ell_I/1

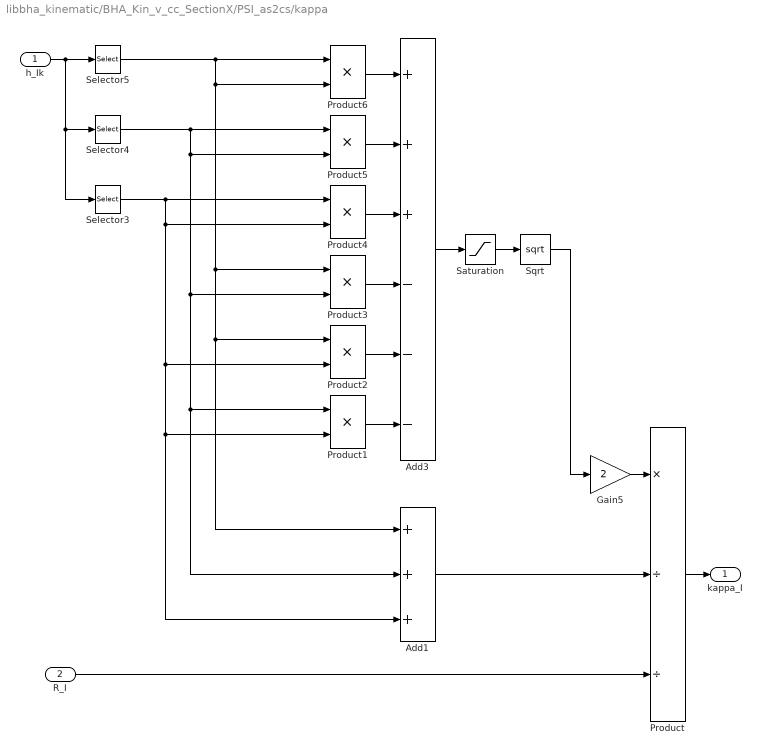
== system libbha_kinematic/BHA_Kin_v_cc_SectionX/PSI_as2cs/kappa ==
  h_Ik : Inport
  R_I : Inport  Port=2
  Add1 : Sum  Inputs=+++
  Add3 : Sum  Inputs=+++---
  Gain5 : Gain  Gain=2
  Product : Product  Inputs=*//  RndMeth=Zero
  Product{1..6} (6 alike) : Product  RndMeth=Zero
  Saturation : Saturate  UpperLimit=inf  LowerLimit=0
  Selector3 : Selector  InputPortWidth=3  IndexOptions=Index vector (dialog)  Indices=3  OutputSizes=1
  Selector4 : Selector  InputPortWidth=3  IndexOptions=Index vector (dialog)  Indices=2  OutputSizes=1
  Selector5 : Selector  InputPortWidth=3  IndexOptions=Index vector (dialog)  Indices=1  OutputSizes=1
  Sqrt : Sqrt  SaturateOnIntegerOverflow=on
  kappa_I : Outport
  wires:
  Selector3/1 -> Add1/3, Product1/2, Product2/2, Product4/2, Product4/1
  Selector4/1 -> Add1/2, Product1/1, Product3/2, Product5/2, Product5/1
  Selector5/1 -> Add1/1, Product2/1, Product3/1, Product6/2, Product6/1
  Saturation/1 -> Sqrt/1
  Gain5/1 -> Product/1
  Sqrt/1 -> Gain5/1
  h_Ik/1 -> Selector3/1, Selector4/1, Selector5/1
  Product6/1 -> Add3/1
  Product5/1 -> Add3/2
  Product4/1 -> Add3/3
  Product3/1 -> Add3/4
  Product2/1 -> Add3/5
  Product1/1 -> Add3/6
  Add3/1 -> Saturation/1
  Add1/1 -> Product/2
  R_I/1 -> Product/3
  Product/1 -> kappa_I/1

== system libbha_kinematic/BHA_Kin_v_cc_SectionX/PSI_as2cs/phi ==
  h_Ik : Inport
  Add : Sum  Inputs=+-
  Add1 : Sum  Inputs=++-
  Gain : Gain  Gain=2
  Gain1 : Gain  Gain=sqrt(3)
  Selector3 : Selector  InputPortWidth=3  IndexOptions=Index vector (dialog)  Indices=3  OutputSizes=1
  Selector4 : Selector  InputPortWidth=3  IndexOptions=Index vector (dialog)  Indices=2  OutputSizes=1
  Selector5 : Selector  InputPortWidth=3  IndexOptions=Index vector (dialog)  Indices=1  OutputSizes=1
  Trigonometric Function : Trigonometry  Operator=atan2
  phi_I : Outport
  wires:
  h_Ik/1 -> Selector5/1, Selector4/1, Selector3/1
  Gain1/1 -> Trigonometric Function/1
  Gain/1 -> Add1/3
  Selector5/1 -> Gain/1
  Add1/1 -> Trigonometric Function/2
  Selector4/1 -> Add1/2, Add/2
  Selector3/1 -> Add1/1, Add/1
  Add/1 -> Gain1/1
  Trigonometric Function/1 -> phi_I/1

== matlab function libbha_kinematic/BHA_Kin_NumDiff_1stO_CC_cont/Zentraler Differenzenquotient -> Jacobimatrix/htH+ ==
  data: h_toolbase input; H_tool input; h output
function h = htH(h_toolbase,H_tool)
    h = H2h(h2H(h_toolbase)*H_tool);
end

function H = h2H(h)
    H= [[h(1:3), h(4:6), h(7:9), h(10:12)]; [0 0 0 1]];
end

function h = H2h(H)
         h = [H(1:3,1);
         H(1:3,2);
         H(1:3,3);
         H(1:3,4)];
end

== matlab function libbha_kinematic/BHA_Kin_DirDiff_1stO_ExtFixedTool ==
  data: H_tool input; h_toolbase input; J_allg_toolbase input; h output; J_allg output
function [h, J_allg]   = Jacobi_CC_continuum(H_tool, h_toolbase, J_allg_toolbase)
n = 3;
% XXXXXXXXXXXXXXXXXXXXXXXXXXXXXXXXXXXXXXXXXXXXXXXXXXXXXXXXXXXXXXXXXXXXXXXXX
% Analytische Berechnung der Jacobi-Matrix J_general bei Verwendung einer
% zusätzlichen konstanten Handachse
% - Modell - Constant Curvature Continuum
%
% Ansatz:
% h = h_general ** H                    ** ist hierbei die Matrizenmultiplikation der homogenen Matrizen. h muss zuvor in H konvertiert werden
% J_general_toolbase = J_general ** H
%
% mit:
% h     = [ H_1,1,  H_2,1,  H_3,1,  H_1,2,  H_2,2,  H_3,2,  H_1,3,  H_2,3,  H_3,3,  H_1,4,  H_2,4,  H_3,4]
%           1       2       3       4       5       6       7       8       9       10      11      12   
%
% Input:
%   H_tool               [4x4]   Homogene Transformation: Koordinatensystem TCP
%                                relativ zum Werkzeugansatz
%   h_toolbase           [12x1]  Pose des Werkzeugansatzes (Homogene Transformation in Vektor geschrieben, ohne Zeile 0,0,0,1)
%   J_allg_toolbase      [12x3n] Jacobi-Matrix des Werkzeugansatzes
%
% Output:
%   h                    [12x1]  Pose des TCP (Homogene Transformation in Vektor geschrieben, ohne Zeile 0,0,0,1)
%   J_allg               [12x3n] Allgemeingültige Jacobi-Matrix für kontinuierliche Manipulatoren
%
% Parameter:
%   n                    [1x1]   Anzahl der Sektionen
%
% Stand: 10.04.2013      Valentin Falkenhahn
% XXXXXXXXXXXXXXXXXXXXXXXXXXXXXXXXXXXXXXXXXXXXXXXXXXXXXXXXXXXXXXXXXXXXXXXXX

    % J_general   = zeros(12, 3*n);
    
    h = htH(h_toolbase,H_tool);
    J_allg = JT(n,J_allg_toolbase,H_tool);

end

function J_general = JT(n,J_general_toolbase,H_tool)

    J_general = zeros(12, 3*n);
    for i=1:3*n
       J_general(:,i) =  htH(J_general_toolbase(:,i),H_tool);
    end

end

% XXXXXXXXXXXXXXXXXXXXXXXXXXXXXXX HELPER XXXXXXXXXXXXXXXXXXXXXXXXXXXXXXXXX

function res = htH(h1,H)
    res = H2h(h2H(h1)*H);
end

function H = h2H(h)
    H= [[h(1:3), h(4:6), h(7:9), h(10:12)]; [0 0 0 1]];
end

function h = H2h(H)
         h = [H(1:3,1);
         H(1:3,2);
         H(1:3,3);
         H(1:3,4)];
end

== matlab function libbha_kinematic/BHA_Kin_NumDiff_1stO_CC_cont/Zentraler Differenzenquotient -> Jacobimatrix/htH- ==
  data: h_toolbase input; H_tool input; h output
function h = htH(h_toolbase,H_tool)
    h = H2h(h2H(h_toolbase)*H_tool);
end

function H = h2H(h)
    H= [[h(1:3), h(4:6), h(7:9), h(10:12)]; [0 0 0 1]];
end

function h = H2h(H)
         h = [H(1:3,1);
         H(1:3,2);
         H(1:3,3);
         H(1:3,4)];
end

== matlab function libbha_kinematic/BHA_Kin_v_cc_SectionX/PSI_cs2ts ==
  data: phi_I input; S_Ih_Ib output; kappa_I input; ell_I input; ell_Ib input; ell_Ih input
function S_Ih_Ib = PSI_cs2ts(phi_I, kappa_I, ell_I, ell_Ib, ell_Ih)

% Berechnung der homogenen Transformation der I-ten Sektion gemäß Abbildung
% PSI_cs2ts(phi_I, kappa_I, ell_I)
% 
% Input:    Konfigurationszustand
% Output:   homogene Transformation zwischen Kopf- und Fuß-Koordinatensystem

%% homogene Transformation des Fußes
U_I0_Ib = [eye(3), [0; 0; ell_Ib];...
           0,0,0,  1];

%% homogene Transformation des Kopfs
U_Ih_I1 = [eye(3), [0; 0; ell_Ih];...
           0,0,0,  1];

%% homogene Transformation des Aktorbereichs
eps =   1e-7;

% Berechnung gemäß lim kappa->0 (Biegelinie ist eine Gerade)
if(kappa_I < eps)
    C_I1_I0 = eye(3);
    O_I1_I0 = [0; 0; ell_I];

% Berechnung gemäß kappa>0 (Biegelinie ist ein Kreissegment)
else
    s_phi   = sin(phi_I);
    c_phi   = cos(phi_I);
    s_kl    = sin(kappa_I*ell_I);
    c_kl    = cos(kappa_I*ell_I);
    
    C_I1_I0 = [c_phi^2*(c_kl-1)+1,      s_phi*c_phi*(c_kl-1),       c_phi*s_kl;...
               s_phi*c_phi*(c_kl-1),    c_phi^2*(1-c_kl)+c_kl,      s_phi*s_kl;...
               -c_phi*s_kl,             -s_phi*s_kl,                c_kl];
           
    O_I1_I0 = [c_phi*(1-c_kl)/kappa_I;...
               s_phi*(1-c_kl)/kappa_I;...
               s_kl/kappa_I];
end
U_I1_I0 = [C_I1_I0, O_I1_I0;...
           0,0,0,   1];
       
S_Ih_Ib = U_I0_Ib*U_I1_I0*U_Ih_I1;

== matlab function libbha_kinematic/BHA_Kin_v_tp_SectionX/Kin_v_Modul ==
  data: l_Ik input; S_lh_lb output; m_I input; a_I0 input; a_Im input; l_Ib input; l_Ih input; theta_I input
function S_lh_lb = ModuleKinematics(l_Ik, m_I, a_I0, a_Im, l_Ib, l_Ih, theta_I)
% l_Ik = Laenge der k Aktoren von Sektion I (NICHT L_Ik gemessene Seillänge incl. base und head)

    % Parameter
    PAR_I.m_I     = m_I;
    PAR_I.a_I0    = a_I0;
    PAR_I.a_Im    = a_Im;
    PAR_I.l_Ib    = l_Ib;
    PAR_I.l_Ih    = l_Ih;
    PAR_I.theta_I = theta_I;
    
    S_lh_lb = mk_l(l_Ik, PAR_I);
end

%% Module-kinematics
function S_lh_lb = mk_l(l_Ik, PAR_I)
    mgl = 0;
    if mgl == 1
        [D_I, N_I_y, Phi_I] = mk_Trafo_l2js(l_Ik, PAR_I);
        [S_lh_lb]         = mk_js(D_I, N_I_y, Phi_I, PAR_I);
    else
        %% Aufbau der Vorwärtskinematik des Base Elements
        h_Ib      = PAR_I.l_Ib*cos(PAR_I.theta_I);
        M_KI0_KIb = [1, 0, 0, 0;...
                     0, 1, 0, 0;...
                     0, 0, 1, h_Ib;...
                     0, 0, 0, 1];

        %% Aufbau der Vorwärtskinematik des Head Elements
        h_Ih      = PAR_I.l_Ih*cos(PAR_I.theta_I);
        M_KIh_KIm = [1, 0, 0, 0;...
                     0, 1, 0, 0;...
                     0, 0, 1, h_Ih;...
                     0, 0, 0, 1];

        %% Aufbau der Vorwärtskinematik des Aktor Elements
        M_KIm_KI0  = eye(4);

        l_IJk = l_Ik / PAR_I.m_I;
        for jj = 1:PAR_I.m_I
            S_KIJ_KIJm = sk_l(l_IJk, jj, PAR_I);
            M_KIm_KI0  = M_KIm_KI0 * S_KIJ_KIJm;
        end

        %% Aufbau der Vorwärtskinematik des gesamten Moduls I
        S_lh_lb = M_KI0_KIb * M_KIm_KI0 * M_KIh_KIm;
    end
end

function S_lh_lb = mk_js(D_I, N_I_y, Phi_I, PAR_I)
    %% Aufbau der Vorwärtskinematik des Base Elements
    h_Ib      = PAR_I.l_Ib*cos(PAR_I.theta_I);
    M_KI0_KIb = [1, 0, 0, 0;...
                 0, 1, 0, 0;...
                 0, 0, 1, h_Ib;...
                 0, 0, 0, 1];

    %% Aufbau der Vorwärtskinematik des Head Elements
    h_Ih      = PAR_I.l_Ih*cos(PAR_I.theta_I);
    M_KIh_KIm = [1, 0, 0, 0;...
                 0, 1, 0, 0;...
                 0, 0, 1, h_Ih;...
                 0, 0, 0, 1];

    %% Aufbau der Vorwärtskinematik des Aktor Elements
    M_KIm_KI0  = eye(4);

    for jj = 1:PAR_I.m_I
        a_IJ  = PAR_I.a_I0-(PAR_I.a_I0-PAR_I.a_Im) * jj/PAR_I.m_I;
        S_KIJ_KIJm = sk_js(D_I, N_I_y, Phi_I/a_IJ, jj, PAR_I);
        M_KIm_KI0  = M_KIm_KI0 * S_KIJ_KIJm;
    end

    %% Aufbau der Vorwärtskinematik des gesamten Moduls I
    S_lh_lb = M_KI0_KIb * M_KIm_KI0 * M_KIh_KIm;
end

function [D_I, N_I_y, Phi_I] = mk_Trafo_l2js(l_Ik, PAR_I)
    %% Berechnung des Gelenkzustands eines Moduls auf Basis des 1. Segments
    l_IJk = l_Ik / PAR_I.m_I;

    [d_I1, n_I1_y, phi_I1] = sk_Trafo_l2js(l_IJk, 1, PAR_I);

    a_I1    = PAR_I.a_I0-(PAR_I.a_I0-PAR_I.a_Im) * 1/PAR_I.m_I;
    
    D_I     = d_I1;
    N_I_y   = n_I1_y;
    Phi_I   = a_I1*phi_I1;
end


%% Segment-kinematics
function S_Kij_Kijm = sk_l(l_IJk, jj, PAR_I)
    [d_IJ, n_IJ_y, phi_IJ] = sk_Trafo_l2js(l_IJk, jj, PAR_I);
    S_Kij_Kijm = sk_js(d_IJ, n_IJ_y, phi_IJ, PAR_I);
end

function S_Kij_Kijm = sk_js(d_ij, n_ij_y, phi_ij, jj, PAR_I)

    s       = sin(phi_ij);
    c       = cos(phi_ij);
    n_ij_x  = sqrt(min(1, max(0, 1-n_ij_y^2)));  % Numerik Absicherung

    S_Kij_Kijm = [c+n_ij_x^2*(1-c),     n_ij_x*n_ij_y*(1-c),    n_ij_y*s,       0;...
                  n_ij_x*n_ij_y*(1-c),  c+n_ij_y^2*(1-c),       -n_ij_x*s,      0;...
                  -n_ij_y*s,            n_ij_x*s,               c,              d_ij;...
                  0,                    0,                      0,              1];

end

function [d_IJ, n_IJ_y, phi_IJ] = sk_Trafo_l2js(l_IJk, jj, PAR_I)
    % Berechnung der Radien der Seilführungen
    a_IJm   = PAR_I.a_I0-(PAR_I.a_I0-PAR_I.a_Im) * (jj-1)/PAR_I.m_I;
    a_IJ    = PAR_I.a_I0-(PAR_I.a_I0-PAR_I.a_Im) * jj/PAR_I.m_I;

    % Berechnung der linearisierten, projizierten Segmentseillängen 
    h_IJk   = sqrt(l_IJk.^2 - ones(3,1)*(a_IJ-a_IJm).^2);

    % Lösung
    d_IJ    = 1/3*sum(h_IJk);
    if(h_IJk(2)-h_IJk(3)~=0)
        if(-2*h_IJk(1)+h_IJk(2)+h_IJk(3)~=0)
            sgn = sign((h_IJk(2)-h_IJk(3))/(-2*h_IJk(1)+h_IJk(2)+h_IJk(3)));
            n_IJ_y = sgn * 1/2 * abs(-2*h_IJk(1)+h_IJk(2)+h_IJk(3))/...
                     sqrt(abs(h_IJk(1)^2+h_IJk(2)^2+h_IJk(3)^2-h_IJk(1)*h_IJk(2)-h_IJk(1)*h_IJk(3)-h_IJk(2)*h_IJk(3)));
        else
            n_IJ_y = 0;
        end
    else
        n_IJ_y = 1;
    end
    n_IJ_y  = max(-1, min(1, n_IJ_y)); %Behebung von Numerikproblem |n_jy| > 1 trotz Einheitsvektor
    n_IJ_x  = sqrt(1-n_IJ_y^2);
    phi_IJ  = -2*(h_IJk(1)-2*h_IJk(2)+h_IJk(3)) / (3*a_IJ.*(n_IJ_y+sqrt(3)*n_IJ_x));
end
